simulink model "rocky_no_motor_feedback"  (R2022b)
settings: Solver=VariableStepAuto  StartTime=0.0  StopTime=10.0  RelTol=1e-3
values from neighbouring files (symbols this model uses):
  a = 13.8265132822    [MotorParams.mat]    (also in Rocky_5_closed_loop_poles.m = 13.8265; Rocky_closed_loop_poles_23.m = 13.83; poles_impulse_step.m = 13.83)
  b = 0.0036184905593    [MotorParams.mat]    (also in Rocky_5_closed_loop_poles.m = 0.0036; Rocky_closed_loop_poles_23.m = 0.0036; poles_impulse_step.m = 0.0036)
  g = 9.81    [RockyParams.mat]    (also in Rocky_5_closed_loop_poles.m; Rocky_closed_loop_poles_23.m; poles_impulse_step.m)
  Ki = 107080    [ControlCoeffs.mat]    (also in Rocky_5_closed_loop_poles.m = real(Ki); Rocky_closed_loop_poles_23.m = double(solutions.Ki); poles_impulse_step.m = double(solutions.Ki))
  Kp = 21242    [ControlCoeffs.mat]    (also in Rocky_5_closed_loop_poles.m = real(Kp); Rocky_closed_loop_poles_23.m = double(solutions.Kp); poles_impulse_step.m = double(solutions.Kp))
  l = 0.436    [RockyParams.mat]    (also in Rocky_5_closed_loop_poles.m; Rocky_closed_loop_poles_23.m; poles_impulse_step.m)
libraries: slpidlib x1
settings Model: Creator=eabbot  LastModifiedBy=eabbot

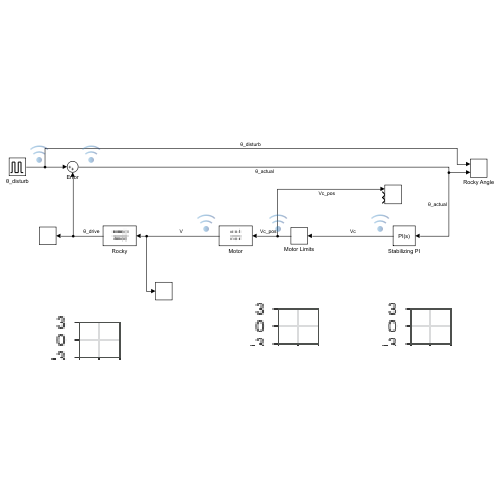
[thumbnail: Simulink's stored preview of the top-level diagram]
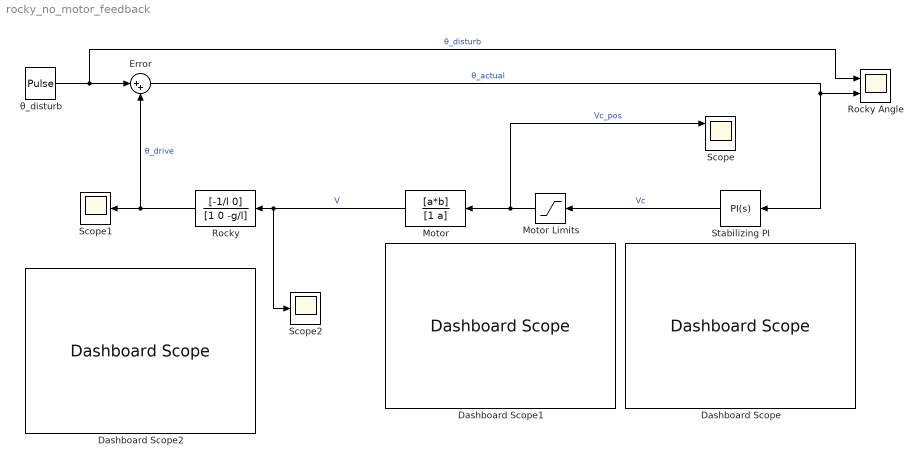
== system rocky_no_motor_feedback ==
  Dashboard Scope : DashboardScope
  Dashboard Scope1 : DashboardScope
  Dashboard Scope2 : DashboardScope
  Error : Sum  Inputs=|++
  Motor : TransferFcn  Numerator=[a*b]  Denominator=[1 a]
  Motor Limits : Saturate  UpperLimit=300  LowerLimit=-300  LinearizeAsGain=off  ZeroCross=off
  Rocky : TransferFcn  Numerator=[-1/l 0]  Denominator=[1 0 -g/l]
  Rocky Angle : Scope  NumInputPorts=2
  Scope : Scope  NumInputPorts=3
  Scope1 : Scope
  Scope2 : Scope
  Stabilizing PI : slpidlib/PID Controller  Controller=PI  Form=Parallel  TimeDomain=Continuous-time  UseExternalTs=off  SampleTime=-1  IntegratorMethod=Forward Euler  FilterMethod=Forward Euler  ControllerParametersSource=internal  P=Kp  I=Ki  UseKiTs=off  D=0  N=100  UseFilter=on  TunerSelectOption=Transfer Function Based (PID Tuner App)  InitialConditionSource=internal  InitialConditionForIntegrator=0  InitialConditionForFilter=0  DifferentiatorICPrevScaledInput=0  ExternalReset=none  TrackingMode=off  Kt=1  LimitOutput=off  SatLimitsSource=internal  UpperSaturationLimit=inf  LowerSaturationLimit=-inf  LinearizeAsGain=on  AntiWindupMode=none  Kb=1  LimitIntegrator=off  UpperIntegratorSaturationLimit=inf  LowerIntegratorSaturationLimit=-inf  POutMin=[]  POutMax=[]  IOutMin=[]  IOutMax=[]  DOutMin=[]  DOutMax=[]  NOutMin=[]  NOutMax=[]  SumOutMin=[]  SumOutMax=[]  SaturationOutMin=[]  SaturationOutMax=[]  PParamMin=[]  PParamMax=[]  IParamMin=[]  IParamMax=[]  DParamMin=[]  DParamMax=[]  NParamMin=[]  NParamMax=[]  KbParamMin=[]  KbParamMax=[]  KtParamMin=[]  KtParamMax=[]  KbOutMin=[]  KbOutMax=[]  KtOutMin=[]  KtOutMax=[]  IntegratorOutMin=[]  IntegratorOutMax=[]  FilterOutMin=[]  FilterOutMax=[]  SumI1OutMin=[]  SumI1OutMax=[]  SumI2OutMin=[]  SumI2OutMax=[]  SumI3OutMin=[]  SumI3OutMax=[]  SumI4OutMin=[]  SumI4OutMax=[]  SumDOutMin=[]  SumDOutMax=[]  DifferentiatorOutMin=[]  DifferentiatorOutMax=[]  FilterDiffOutCoefMin=[]  FilterDiffOutCoefMax=[]  ReciprocalOutMin=[]  ReciprocalOutMax=[]  SumDenOutMin=[]  SumDenOutMax=[]  SumNumOutMin=[]  SumNumOutMax=[]  DivideOutMin=[]  DivideOutMax=[]  UdiffTsProdOutMin=[]  UdiffTsProdOutMax=[]  NTsProdOutMin=[]  NTsProdOutMax=[]  UintegralTsProdOutMin=[]  UintegralTsProdOutMax=[]  UngainTsProdOutMin=[]  UngainTsProdOutMax=[]  ClampingZeroOutDataTypeStr=Inherit: Inherit via back propagation  ClampingZeroOutMin=[]  ClampingZeroOutMax=[]  FilterDenConstantOutDataTypeStr=Inherit: Inherit via back propagation  FilterDenConstantOutMin=[]  FilterDenConstantOutMax=[]  PCopyOutDataTypeStr=Inherit: Inherit via back propagation  PCopyOutMin=[]  PCopyOutMax=[]  NCopyOutDataTypeStr=Inherit: Inherit via back propagation  NCopyOutMin=[]  NCopyOutMax=[]  IntegratorContinuousStateAttributes=''  IntegratorStateMustResolveToSignalObject=off  IntegratorRTWStateStorageClass=Auto  FilterContinuousStateAttributes=''  FilterStateMustResolveToSignalObject=off  FilterRTWStateStorageClass=Auto  ParallelPVariant=InternalParameters  IdealPVariant=Disabled  IVariant=InternalParameters  DVariant=Disabled  IntegratorVariant=Continuous  SatVariant=Disabled  AWVariant=Passthrough  PCopyVariant=Disabled  TRVariant=Disabled  FdbkBlocksVariant=Forward  IdealPFdbkVariant=Disabled  SatFdbkVariant=Disabled  DerivativeFilterVariant=Disabled  NVariant=Disabled  NCopyVariant=Disabled_SignalSpec  FilterICVariant=Disabled  IntegratorICVariant=InternalICs  ExternalResetVariant=Disabled  TRSumVariant=Passthrough  SumFdbkVariant=Disabled  SumVariant=Sum_PI  TsampFilterVariant=InternalTs  TsampNgainVariant=Passthrough  TsampIntegralVariant=Passthrough  ExternalSaturationOutDataTypeStr=Inherit: Same as second input
  θ_disturb : DiscretePulseGenerator  PulseType=Time based  Amplitude=0.1  Period=4  PulseWidth=0.5
  wires:
  Stabilizing PI/1 -> Motor Limits/1  "Vc"
  Rocky/1 -> Scope1/1, Error/2  "θ_drive"
  Error/1 -> Stabilizing PI/1, Rocky Angle/2  "θ_actual"
  Motor/1 -> Scope2/1, Rocky/1  "V"
  Motor Limits/1 -> Scope/1, Motor/1  "Vc_pos"
  θ_disturb/1 -> Rocky Angle/1, Error/1  "θ_disturb"
